simulink model "simulation_ex_3_2014a"  (R2014a)
settings: Solver=ode45  SolverMode=SingleTasking  StartTime=0.0  StopTime=10  RelTol=1e-3
settings Model: CovMetricSettings=dwe  CovHtmlReporting=off  covSaveCumulativeToWorkspaceVar=off  CovSaveSingleToWorkspaceVar=off  CovExternalEMLEnable=on  CovSFcnEnable=on  Creator=HanO  LastModifiedBy=HanO
settings DataIOCC: LimitDataPoints=off  SaveFormat=StructureWithTime  ReturnWorkspaceOutputs=on
settings DebuggingCC: MergeDetectMultiDrivingBlocksExec=error  SolverPrmCheckMsg=none  FrameProcessingCompatibilityMsg=error  SFUnexpectedBacktrackingDiag=error  SFNoUnconditionalDefaultTransitionDiag=error
settings HardwareCC: ProdBitPerPointer=64  ProdLargestAtomicFloat=Float  ProdIntDivRoundTo=Zero  ProdEndianess=LittleEndian  ProdHWDeviceType=Specified
settings ModelReferenceCC: PropagateSignalLabelsOutOfModel=on
settings SFSimCC: SimUseLocalCustomCode=on
settings RTWCC: RTWUseLocalCustomCode=on
settings GRTTargetCC: TargetLangStandard=C99 (ISO)

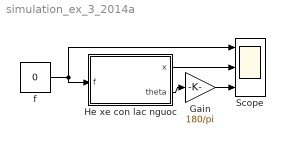
== system simulation_ex_3_2014a ==
  Gain : Gain  Gain=180/pi
  He xe con lac nguoc : Subsystem  mask{MM=2, m=0.1, l=0.5, g=9.81, x0=10, theta0=pi/2}
      mask prompts: MM "Khối lượng xe M"; m "Khối lượng vật nặng đầu con lắc m"; l "Chiều dài con lắc l"; g "Gia tốc trọng trường g"; x0 "Vị trí ban đầu của xe x0"; theta0 "Góc lệch ban đầu của con lắc theta0"
  Scope : Scope  NumInputPorts=3
      settings: TimeRange=auto  MaxDataPoints=5000  SaveName=ScopeData  YMin=-1.00000~9.99285~67.51929  YMax=1.00000~10.05374~292.32637  SampleTime=-1
  f : Constant  Value=0
  wires:
  f/1 -> Scope/1, He xe con lac nguoc/1(f)
  He xe con lac nguoc/1(x) -> Scope/2
  He xe con lac nguoc/2(theta) -> Gain/1
  Gain/1 -> Scope/3

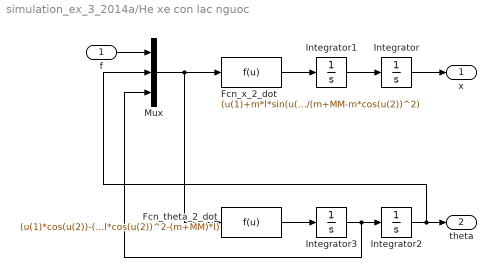
== system simulation_ex_3_2014a/He xe con lac nguoc ==
  f : Inport
  Fcn_theta_2_dot : Fcn  Expr=(u(1)*cos(u(2))-(m+MM)*g*sin(u(2))+m*l*sin(u(2))*cos(u(2))*u(3)^2)/(m*l*cos(u(2))^2-(m+MM)*l)
  Fcn_x_2_dot : Fcn  Expr=(u(1)+m*l*sin(u(2))*u(3)^2-m*g*sin(u(2))*cos(u(2)))/(m+MM-m*cos(u(2))^2)
  Integrator : Integrator  InitialCondition=x0
  Integrator1 : Integrator
  Integrator2 : Integrator  InitialCondition=theta0
  Integrator3 : Integrator
  Mux : Mux  Inputs=3
  x : Outport
  theta : Outport  Port=2
  wires:
  Integrator1/1 -> Integrator/1
  Integrator/1 -> x/1
  Fcn_x_2_dot/1 -> Integrator1/1
  Fcn_theta_2_dot/1 -> Integrator3/1
  Mux/1 -> Fcn_theta_2_dot/1, Fcn_x_2_dot/1
  f/1 -> Mux/1
  Integrator2/1 -> Mux/2, theta/1
  Integrator3/1 -> Mux/3, Integrator2/1
